simulink model "Smart_City_QCar2_calibrate_r2020a"  (R2020a)
settings: Solver=ode1  StartTime=0.0  StopTime=10  FixedStep=1/20  RelTol=1e-3  EnableMultiTasking=on
undefined symbols (not defined in the file): Point
libraries: quarc_library x4
settings Model: SimulationMode=external  ExtModeTrigDuration=10000  Creator=PKaram  LastModifiedBy=user
settings SolverCC: PositivePriorityOrder=on  AutoInsertRateTranBlk=on
settings DataIOCC: ReturnWorkspaceOutputs=off
settings DebuggingCC: ParameterPrecisionLossMsg=none  ArithmeticOperatorsInVariantConditions=warning
settings HardwareCC: ProdBitPerLong=64  ProdLargestAtomicInteger=LongLong  ProdLargestAtomicFloat=Double  ProdLongLongMode=on  ProdHWDeviceType=ARM Compatible->ARM 64-bit (LP64)
settings SFSimCC: SimUseLocalCustomCode=off  CustomCodeUndefinedFunction=UseInterfaceOnly
settings RTWCC: Description=QUARC Linux QCar2 Target Using Toolchain  SystemTargetFile=quarc_linux_qcar2.tlc  TemplateMakefile=quarc_linux_nvidia_tmf  RTWUseLocalCustomCode=off  Toolchain=QUARC linux_qcar2 | gmake (64-bit Windows)  BuildConfiguration=Faster Runs
settings CodeAppCC: StateflowObjectComments=on
settings STFCustomTargetCC: TargetLangStandard=C99 (ISO)  ConcurrentExecutionCompliant=on  GRTInterface=on  UseToolchainInfoCompliant=on  SystemTargetFile=quarc_linux_qcar2.tlc
settings GRTTargetCC: ParMdlRefBuildCompliant=off  CompOptLevelCompliant=off  CombineOutputUpdateFcns=off  MatFileLogging=off  CPPClassGenCompliant=off  GRTInterface=on  ExtMode=on  ExtModeMexFile=quarc_comm  ExtModeMexArgs='-w -d /home/nvidia/Documents -uri %u', 'tcpip://192.168.2.14:17001'
settings ConfigComp: CovMetricSettings=dswe

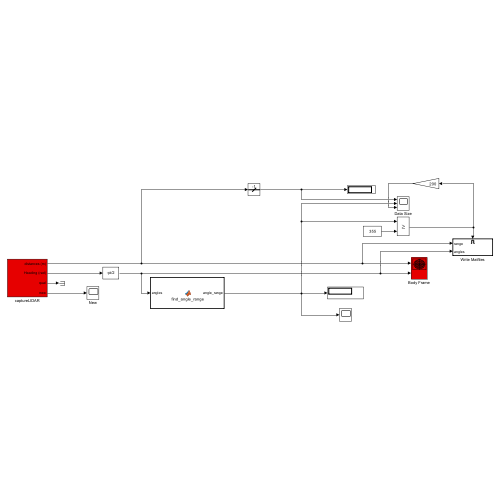
[thumbnail: Simulink's stored preview of the top-level diagram]
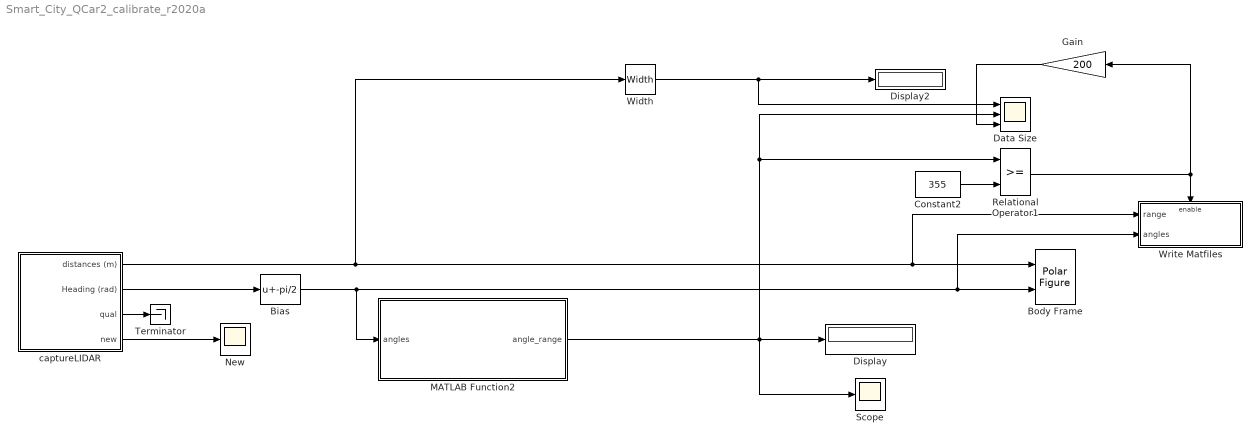
== system Smart_City_QCar2_calibrate_r2020a ==
  Bias : Bias  Bias=-pi/2
  Body Frame : quarc_library/Sinks/Figures/Polar Figure  figure_mode=Use figure window  figure_tag=figure1  axes_tag=axes1  plot_mode=Frame-based  minimum_rho=0  maximum_rho=7  minimum_theta=0  maximum_theta=360  zero_location=right  direction=clockwise  buffer_size=1000  update_rate=1  sample_time=-1  initial_position="2    41  1918   982"  initial_visibility=off  line1_style=None  line1_width=0.5  line1_color=[0 0.4470 0.7410]  marker1=Point (.)  marker1_size=1  marker1_edge_color=[0 0.447059 0.741176]  marker1_face_color=[0 0.447059 0.741176]  line2_style=Solid line (-)  line2_width=0.5  line2_color=[0.85098 0.32549 0.0980392]  marker2=None  marker2_size=6  marker2_edge_color=[0.85098 0.32549 0.0980392]  marker2_face_color=[0.85098 0.32549 0.0980392]  line3_style=Solid line (-)  line3_width=0.5  line3_color=[0.929412 0.694118 0.12549]  marker3=None  marker3_size=6  marker3_edge_color=[0.929412 0.694118 0.12549]  marker3_face_color=[0.929412 0.694118 0.12549]  line4_style=Solid line (-)  line4_width=0.5  line4_color=[0.494118 0.184314 0.556863]  marker4=None  marker4_size=6  marker4_edge_color=[0.494118 0.184314 0.556863]  marker4_face_color=[0.494118 0.184314 0.556863]  line5_style=Solid line (-)  line5_width=0.5  line5_color=[0.466667 0.67451 0.188235]  marker5=None  marker5_size=6  marker5_edge_color=[0.466667 0.67451 0.188235]  marker5_face_color=[0.466667 0.67451 0.188235]
      settings: SourceProductName=QUARC Targets
  Constant2 : Constant  Value=355
  Data Size : Scope  NumInputPorts=3
  Display : Display
  Display2 : Display
  Gain : Gain  Gain=200
  MATLAB Function2 : MATLAB Function  TreatAsAtomicUnit=on
  New : Scope
  Relational Operator1 : RelationalOperator  OutDataTypeStr=boolean  RndMeth=Simplest
  Scope : Scope
  Terminator : Terminator
  Width : Width
  Write Matfiles : Subsystem  TreatAsAtomicUnit=on
  captureLIDAR : Subsystem
  wires:
  captureLIDAR/2(Heading (rad)) -> Bias/1
  captureLIDAR/1(distances (m)) -> Write Matfiles/1(range), Body Frame/1, Width/1
  Width/1 -> Display2/1, Data Size/1
  MATLAB Function2/1(angle_range) -> Scope/1, Display/1, Relational Operator1/1, Data Size/2
  Bias/1 -> Write Matfiles/2(angles), Body Frame/2, MATLAB Function2/1(angles)
  Constant2/1 -> Relational Operator1/2
  Gain/1 -> Data Size/3
  captureLIDAR/4(new) -> New/1
  captureLIDAR/3(qual) -> Terminator/1
  Relational Operator1/1 -> Gain/1, Write Matfiles/Enable

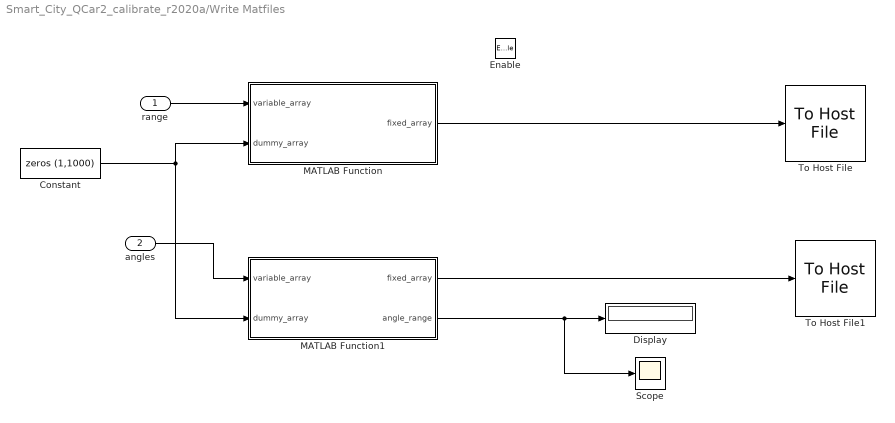
== system Smart_City_QCar2_calibrate_r2020a/Write Matfiles ==
  range : Inport
  angles : Inport  Port=2
  Enable : EnablePort
  Constant : Constant  Value=zeros (1,1000)
  Display : Display
  MATLAB Function : MATLAB Function  TreatAsAtomicUnit=on
  MATLAB Function1 : MATLAB Function  TreatAsAtomicUnit=on
  Scope : Scope
  To Host File : quarc_library/Sinks/To Host/To Host File  source=Specify via dialog (do not evaluate)  file_name=distance_new_qcar2.mat  variable_name=distance_new_qcar2  decimation=1  sample_time=-1  file_format=MAT-file v.4  options=No header or footer  append=off  final_file_name=distance_new_qcar2.mat  encoding=Default  bitrate=2000000
  To Host File1 : quarc_library/Sinks/To Host/To Host File  source=Specify via dialog (do not evaluate)  file_name=angles_new_qcar2.mat  variable_name=angles_new_qcar2  decimation=1  sample_time=-1  file_format=MAT-file v.4  options=No header or footer  append=off  final_file_name=angles_new_qcar2.mat  encoding=Default  bitrate=2000000
  wires:
  range/1 -> MATLAB Function/1(variable_array)
  MATLAB Function/1(fixed_array) -> To Host File/1
  angles/1 -> MATLAB Function1/1(variable_array)
  Constant/1 -> MATLAB Function/2(dummy_array), MATLAB Function1/2(dummy_array)
  MATLAB Function1/1(fixed_array) -> To Host File1/1
  MATLAB Function1/2(angle_range) -> Scope/1, Display/1

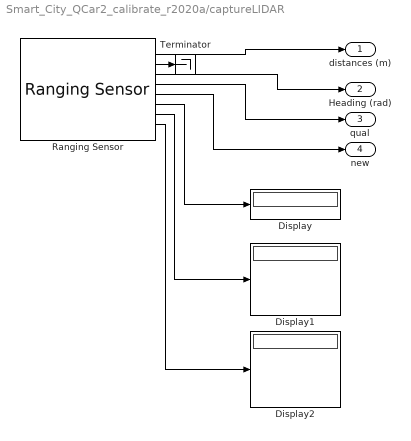
== system Smart_City_QCar2_calibrate_r2020a/captureLIDAR ==
  Display : Display
      settings: Decimation=100
  Display1 : Display
      settings: Decimation=100
  Display2 : Display
      settings: Decimation=100
  Ranging Sensor : quarc_library/Devices/Third-Party/Sensors/Ranging Sensor  sensor_type=RPLidar LIDAR  uri=serial-cpu://localhost:1?baud='256000',word='8',parity='none',stop='1',flow='none',dsr='on'  ranging_distance=Long  timing_budget=0.033  measurement_period=0.040  output_mode=Variable-size output  samples_per_revolution=1000  max_distance=0.050  max_angle=5  sample_time=qc_get_step_size  show_versions=on  active=on
      settings: SourceProductName=QUARC Targets
  Terminator : Terminator
  distances (m) : Outport  VectorParamsAs1DForOutWhenUnconnected=off
  Heading (rad) : Outport  Port=2  VectorParamsAs1DForOutWhenUnconnected=off
  qual : Outport  Port=3  VectorParamsAs1DForOutWhenUnconnected=off
  new : Outport  Port=4  VectorParamsAs1DForOutWhenUnconnected=off
  wires:
  Ranging Sensor/1 -> distances (m)/1
  Ranging Sensor/3 -> Heading (rad)/1
  Ranging Sensor/4 -> qual/1
  Ranging Sensor/5 -> new/1
  Ranging Sensor/6 -> Display/1
  Ranging Sensor/7 -> Display1/1
  Ranging Sensor/8 -> Display2/1
  Ranging Sensor/2 -> Terminator/1

== matlab function Smart_City_QCar2_calibrate_r2020a/MATLAB Function2 ==
  data: angles input; angle_range output
function angle_range = find_angle_range (angles)
angle_range = 0;
angle_range = max (angles) - min(angles);
angle_range = 180/pi*angle_range;

== matlab function Smart_City_QCar2_calibrate_r2020a/Write Matfiles/MATLAB Function1 ==
  data: variable_array input; fixed_array output; dummy_array input; angle_range output
function [fixed_array, angle_range] = make_fixed (variable_array, dummy_array)
fixed_array = dummy_array;
angle_range = 0;
for i = 1:length (variable_array)
    fixed_array(i) = variable_array (i);
end
% angle_range = variable_array(length (variable_array)) - variable_array(1);
angle_range = max (variable_array) - min(variable_array);
angle_range = 180/pi*angle_range;

== matlab function Smart_City_QCar2_calibrate_r2020a/Write Matfiles/MATLAB Function ==
  data: variable_array input; fixed_array output; dummy_array input
function fixed_array = make_fixed (variable_array, dummy_array)
fixed_array = dummy_array;
for i = 1:length (variable_array)
    fixed_array(i) = variable_array (i);
end
